simulink model "RGB_Color_Component_AutoThresholding"  (R2016a)
settings: Solver=VariableStepAuto  StartTime=0.0  StopTime=inf  RelTol=1e-3
undefined symbols (not defined in the file): none, Rec, SDTV, videoinput
libraries: visionstatistics x6, visionconversions x3, visionsinks x2, imaqlib x1
settings Model: Creator=YASARA  LastModifiedBy=YASARA

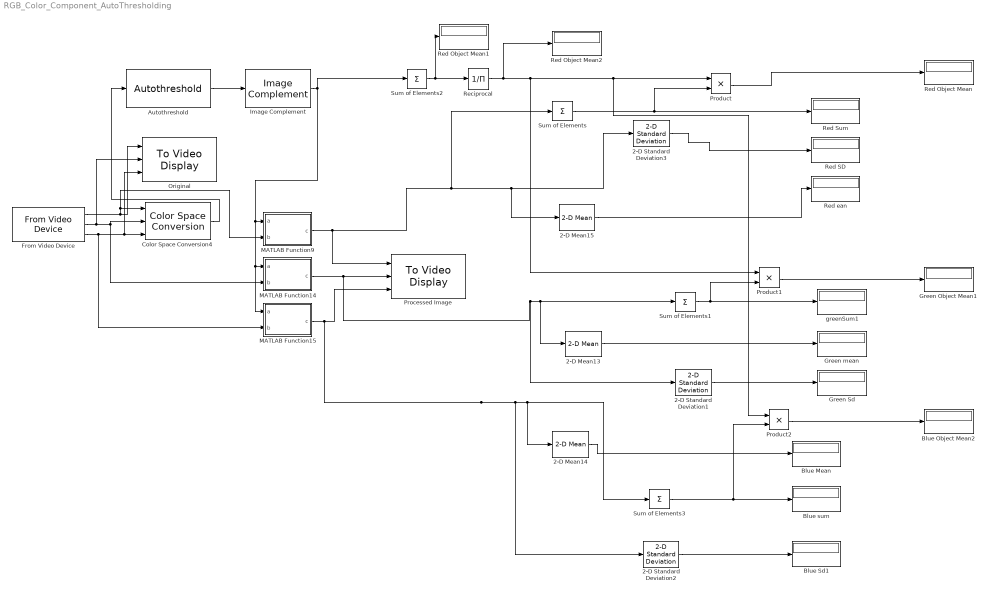
== system RGB_Color_Component_AutoThresholding ==
  2-D Mean13 : visionstatistics/2-D Mean  run=off  reset_popup=None  directionMode=Entire input  dimension=1  treatSBRowAsCol=on  roiEnable=off  roiType=Rectangles  roiPortion=Entire ROI  roiOutput=Individual statistics for each ROI  roiFlag=off  outputDataTypeStr=Inherit: Same as accumulator  outputLastDataTypeStr=Inherit: Same as accumulator  outputMin=[]  outputMax=[]  accumMode=Binary point scaling  accumWordLength=32  accumFracLength=0  accumDataTypeStr=fixdt([],32,0)  accumLastDataTypeStr=fixdt([],32,0)  roundingMode=Floor  overflowMode=off
  2-D Mean14 : visionstatistics/2-D Mean  run=off  reset_popup=None  directionMode=Entire input  dimension=1  treatSBRowAsCol=on  roiEnable=off  roiType=Rectangles  roiPortion=Entire ROI  roiOutput=Individual statistics for each ROI  roiFlag=off  outputDataTypeStr=Inherit: Same as accumulator  outputLastDataTypeStr=Inherit: Same as accumulator  outputMin=[]  outputMax=[]  accumMode=Binary point scaling  accumWordLength=32  accumFracLength=0  accumDataTypeStr=fixdt([],32,0)  accumLastDataTypeStr=fixdt([],32,0)  roundingMode=Floor  overflowMode=off
  2-D Mean15 : visionstatistics/2-D Mean  run=off  reset_popup=None  directionMode=Entire input  dimension=1  treatSBRowAsCol=on  roiEnable=off  roiType=Rectangles  roiPortion=Entire ROI  roiOutput=Individual statistics for each ROI  roiFlag=off  outputDataTypeStr=Inherit: Same as accumulator  outputLastDataTypeStr=Inherit: Same as accumulator  outputMin=[]  outputMax=[]  accumMode=Binary point scaling  accumWordLength=32  accumFracLength=0  accumDataTypeStr=fixdt([],32,0)  accumLastDataTypeStr=fixdt([],32,0)  roundingMode=Floor  overflowMode=off
  2-D Standard Deviation1 : visionstatistics/2-D Standard Deviation  run=off  reset_popup=None  directionMode=Entire input  dimension=1  treatSBRowAsCol=on  roiEnable=off  roiType=Rectangles  roiPortion=Entire ROI  roiOutput=Individual statistics for each ROI  roiFlag=off
  2-D Standard Deviation2 : visionstatistics/2-D Standard Deviation  run=off  reset_popup=None  directionMode=Entire input  dimension=1  treatSBRowAsCol=on  roiEnable=off  roiType=Rectangles  roiPortion=Entire ROI  roiOutput=Individual statistics for each ROI  roiFlag=off
  2-D Standard Deviation3 : visionstatistics/2-D Standard Deviation  run=off  reset_popup=None  directionMode=Entire input  dimension=1  treatSBRowAsCol=on  roiEnable=off  roiType=Rectangles  roiPortion=Entire ROI  roiOutput=Individual statistics for each ROI  roiFlag=off
  Autothreshold : visionconversions/Autothreshold  operator=>  threshOut=off  effMetricOut=off  userDefinedRange=off  umin=0  umax=255  outOfRngOpt=Warn and saturate  scaleThreshold=off  scaleFactor=1  P1Mode=Specify word length  P1WordLength=32  P1FracLength=30  P2Mode=Specify word length  P2WordLength=32  P2FracLength=22  P3Mode=Specify word length  P3WordLength=32  P3FracLength=14  P4Mode=Binary point scaling  P4WordLength=32  P4FracLength=15  Q1Mode=Specify word length  Q1WordLength=32  Q1FracLength=16  EMMode=Specify word length  EMWordLength=16  EMFracLength=14  roundingMode=Floor  overflowMode=off
  Blue Mean : Display
  Blue Object Mean2 : Display
  Blue Sd1 : Display
  Blue sum : Display
  Color Space Conversion4 : visionconversions/Color Space  Conversion  conversion=Obsolete  conversionActive=R'G'B' to intensity  wp_str=D65  rec=Rec. 601 (SDTV)  sys=1125/60/2:1  imagePorts=Separate color signals
  From Video Device : imaqlib/From Video Device  DeviceMenu=winvideo 2 (USB Video Device)  Device=winvideo 2 (USB Video Device)  ObjConstructor=videoinput('winvideo', 2)  VideoFormatMenu=YUY2_160x120  VideoFormat=YUY2_160x120  VideoSource=input1  ROIPosition=[0 0 120 160]  EnableHWTrigger=off  TriggerConfiguration=none/none  SampleTime=1/30  OutputPortsMode=Separate color signals  DataType=double  CanDoHWTrigger=no  ReturnedColorSpace=rgb  BlockHandle=44.0042  ROIWidth=160  ROIHeight=120  ROIColumn=0  ROIRow=0  EngXMLPath=C:\Program Files\MATLAB\R2016a\toolbox\imaq\imaq\private  DevXMLPath=C:\MATLAB\SupportPackages\R2016a\toolbox\imaq\supportpackages\genericvideo\adaptor\win64  EngLibPath=C:\Program Files\MATLAB\R2016a\toolbox\imaq\imaqblks\imaqmex\win64  ColorSpace=rgb  BayerSensorAlignment=grbg
  Green Object Mean1 : Display
  Green Sd : Display
  Green mean : Display
  Image Complement : visionconversions/Image Complement
  MATLAB Function14 : MATLAB Function  TreatAsAtomicUnit=on
  MATLAB Function15 : MATLAB Function  TreatAsAtomicUnit=on
  MATLAB Function9 : MATLAB Function  TreatAsAtomicUnit=on
  Original : visionsinks/To Video Display  windowSizeMode=Normal  openAtMdlStart=on  fullScreen=off  videoWindowX=217  videoWindowY=207  saveWindowSize=off  videoWindowWidth=512  videoWindowHeight=384  inputColorFormat=RGB  inputType=Obsolete  imagePorts=Separate color signals  OutputDevice=On-screen video monitor  dataOrg=Column-major  isWindowOpen=off
  Processed Image : visionsinks/To Video Display  windowSizeMode=Normal  openAtMdlStart=on  fullScreen=off  videoWindowX=730  videoWindowY=207  saveWindowSize=off  videoWindowWidth=512  videoWindowHeight=384  inputColorFormat=RGB  inputType=Obsolete  imagePorts=Separate color signals  OutputDevice=On-screen video monitor  dataOrg=Column-major  isWindowOpen=off
  Product : Product
  Product1 : Product
  Product2 : Product
  Reciprocal : Product  Inputs=/  OutDataTypeStr=double  SaturateOnIntegerOverflow=on  RndMeth=Zero
  Red Object Mean : Display
  Red Object Mean1 : Display
  Red Object Mean2 : Display
  Red SD : Display
  Red Sum : Display
  Red ean : Display
  Sum of Elements{,1..3} (4 alike) : Sum  Inputs=+
  greenSum1 : Display
  wires:
  Autothreshold/1 -> Image Complement/1
  Color Space Conversion4/1 -> Autothreshold/1
  2-D Mean15/1 -> Red ean/1
  2-D Mean13/1 -> Green mean/1
  Sum of Elements/1 -> Product/2, Red Sum/1
  MATLAB Function9/1(c) -> Processed Image/1, 2-D Mean15/1, 2-D Standard Deviation3/1, Sum of Elements/1
  2-D Standard Deviation3/1 -> Red SD/1
  2-D Standard Deviation1/1 -> Green Sd/1
  MATLAB Function14/1(c) -> Processed Image/2, 2-D Standard Deviation1/1, 2-D Mean13/1, Sum of Elements1/1
  Sum of Elements3/1 -> Product2/2, Blue sum/1
  2-D Standard Deviation2/1 -> Blue Sd1/1
  MATLAB Function15/1(c) -> Processed Image/3, 2-D Standard Deviation2/1, 2-D Mean14/1, Sum of Elements3/1
  Sum of Elements2/1 -> Red Object Mean1/1, Reciprocal/1
  Product/1 -> Red Object Mean/1
  Sum of Elements1/1 -> Product1/2, greenSum1/1
  Product1/1 -> Green Object Mean1/1
  2-D Mean14/1 -> Blue Mean/1
  Product2/1 -> Blue Object Mean2/1
  Reciprocal/1 -> Red Object Mean2/1, Product2/1, Product/1, Product1/1
  Image Complement/1 -> MATLAB Function15/1(a), MATLAB Function14/1(a), MATLAB Function9/1(a), Sum of Elements2/1
  From Video Device/1 -> Original/1, MATLAB Function9/2(b), Color Space Conversion4/1
  From Video Device/2 -> Original/2, Color Space Conversion4/2, MATLAB Function14/2(b)
  From Video Device/3 -> MATLAB Function15/2(b), Original/3, Color Space Conversion4/3

== matlab function RGB_Color_Component_AutoThresholding/MATLAB Function14 ==
  data: a input; b input; c output
function c = fcn(a,b)
%#codegen
c=a.*b;
return

== matlab function RGB_Color_Component_AutoThresholding/MATLAB Function15 ==
  data: a input; b input; c output
function c = fcn(a,b)
%#codegen
c=a.*b;
return

== matlab function RGB_Color_Component_AutoThresholding/MATLAB Function9 ==
  data: a input; b input; c output
function c = fcn(a,b)
%#codegen
c=a.*b;
return
